simulink model "primary"  (R2017b)
settings: Solver=VariableStepAuto  StartTime=0.0  StopTime=10.0  RelTol=1e-3
model workspace (MAT data in the model file):
  Cf = 0
  F = 0
  Kic = 0
  Kiv = 0
  Kpc = 0
  Kpv = 0
  Lf = 0
  Vn = 0
  fn = 0
  m = 0
  n = 0
  wn = 0
libraries: powerlib x13, powerlib_meascontrol x5, simulink x4, pePowerMeasurement x1
settings Model: Creator=xx  LastModifiedBy=ongun

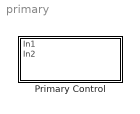
== system primary ==
  Primary Control : Subsystem

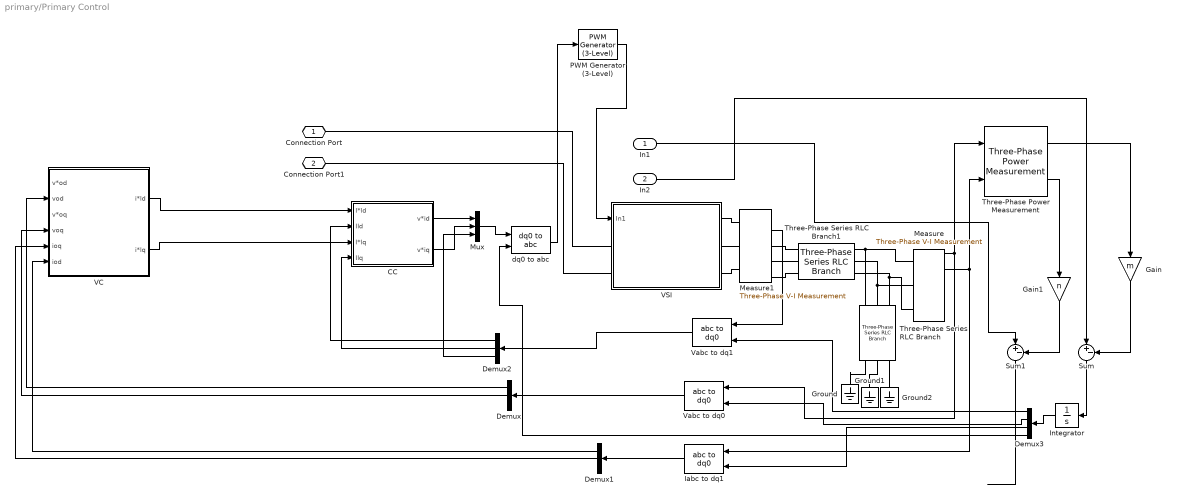
== system primary/Primary Control ==
  In1 : Inport
  In2 : Inport  Port=2
  CC : Subsystem
  Demux : Demux  Outputs=3
  Demux1 : Demux  Outputs=3
  Demux2 : Demux  Outputs=3
  Demux3 : Demux
  Gain : Gain  Gain=m
  Gain1 : Gain  Gain=n
  Ground : powerlib/Elements/Ground  LConnTagsString=a
  Ground1 : powerlib/Elements/Ground  LConnTagsString=a
  Ground2 : powerlib/Elements/Ground  LConnTagsString=a
  Iabc to dq1 : powerlib_meascontrol/Transformations/abc to dq0  Alignment=90 degrees behind phase A axis
  Integrator : Integrator
  Measure : powerlib/Measurements/Three-Phase V-I Measurement  VoltageMeasurement=phase-to-ground  SetLabelV=off  LabelV=V1  Vpu=off  VpuLL=off  CurrentMeasurement=yes  SetLabelI=off  LabelI=I1  Ipu=off  Pbase=5.5e3  Vbase=385  OutputType=Magnitude  PhasorSimulation=off  PSBequivalent=0
  Measure1 : powerlib/Measurements/Three-Phase V-I Measurement  VoltageMeasurement=phase-to-ground  SetLabelV=off  LabelV=V1  Vpu=off  VpuLL=off  CurrentMeasurement=yes  SetLabelI=off  LabelI=I1  Ipu=off  Pbase=5.5e3  Vbase=385  OutputType=Magnitude  PhasorSimulation=off  PSBequivalent=0
  Mux : Mux  Inputs=3
  PWM Generator (3-Level) : powerlib_meascontrol/Pulse & Signal Generators/PWM Generator (3-Level)  ModulatorType=Three-phase bridge (12 pulses)  ModulatorMode=Unsynchronized  nF=27  Fc=27*60  ModulatingSignals=off  m=0.8  Freq=60  Phase=0  Ts=0
      settings: SourceProductName=Simscape Power Systems  SourceProductBaseCode=PS
  Sum : Sum  Inputs=|+-
  Sum1 : Sum  Inputs=|+-
  Three-Phase Series RLC Branch : powerlib/Elements/Three-Phase Series RLC Branch  LConnTagsString=A|B|C  RConnTagsString=A|B|C  BranchType=C  Resistance=.1  Inductance=1e-3  Capacitance=6.85e-6  Measurements=None
  Three-Phase Series RLC Branch1 : powerlib/Elements/Three-Phase Series RLC Branch  LConnTagsString=A|B|C  RConnTagsString=A|B|C  BranchType=RL  Resistance=1  Inductance=1e-3  Capacitance=0  Measurements=None
  Three-Phase Power Measurement : pePowerMeasurement/Three-Phase Power Measurement  OverrideUsingVariant=Continuous  F=60  K=[0 1 2 3]  Seq=Positive  Ts=0
  VC : Subsystem
  VSI : Subsystem
  Vabc to dq0 : powerlib_meascontrol/Transformations/abc to dq0  Alignment=90 degrees behind phase A axis
  Vabc to dq1 : powerlib_meascontrol/Transformations/abc to dq0  Alignment=90 degrees behind phase A axis
  dq0 to abc : powerlib_meascontrol/Transformations/dq0 to abc  Alignment=90 degrees behind phase A axis
  Connection Port : PMIOPort  Port=1  Side=Left
  Connection Port1 : PMIOPort  Port=2  Side=Left
  wires:
  Demux/1 -> VC/2(vod)
  Demux/2 -> VC/4(voq)
  Measure/2 -> Three-Phase Power Measurement/2, Iabc to dq1/1
  Three-Phase Power Measurement/2 -> Gain1/1
  Demux2/2 -> CC/4(Ilq)
  In1/1 -> Sum1/1
  VC/1(i*ld) -> CC/1(I*ld)
  Measure1/2 -> Vabc to dq1/1
  In2/1 -> Sum/1
  Three-Phase Power Measurement/1 -> Gain/1
  Vabc to dq0/1 -> Demux/1
  Vabc to dq1/1 -> Demux2/1
  Gain1/1 -> Sum1/2
  Demux2/1 -> CC/2(Ild)
  Demux1/2 -> VC/5(ioq)
  Measure/1 -> Three-Phase Power Measurement/1, Vabc to dq0/1
  Gain/1 -> Sum/2
  Sum/1 -> Integrator/1
  VC/2("i*lq ") -> CC/3(I*lq)
  Demux1/1 -> VC/6(iod)
  Iabc to dq1/1 -> Demux1/1
  Sum1/1 -> ?
  CC/1(v*id) -> Mux/1
  CC/2("v*iq ") -> Mux/2
  Demux2/3 -> Mux/3
  Mux/1 -> dq0 to abc/1
  dq0 to abc/1 -> PWM Generator (3-Level)/1
  PWM Generator (3-Level)/1 -> VSI/1(In1)
  Integrator/1 -> Demux3/1
  Demux3/3 -> Iabc to dq1/2
  Demux3/2 -> Vabc to dq0/2
  Demux3/1 -> Vabc to dq1/2
  Demux3/4 -> dq0 to abc/2
  connections:
  VSI/RConn2 -- Measure1/LConn2
  VSI/RConn1 -- Measure1/LConn1
  VSI/RConn3 -- Measure1/LConn3
  Connection Port/RConn1 -- VSI/LConn1
  VSI/LConn2 -- Connection Port1/RConn1
  Three-Phase Series RLC Branch/LConn3 -- Measure/LConn3 -- Three-Phase Series RLC Branch1/RConn3
  Three-Phase Series RLC Branch1/RConn1 -- Measure/LConn1 -- Three-Phase Series RLC Branch/LConn1
  Three-Phase Series RLC Branch1/RConn2 -- Measure/LConn2 -- Three-Phase Series RLC Branch/LConn2
  Ground/LConn1 -- Three-Phase Series RLC Branch/RConn1
  Ground1/LConn1 -- Three-Phase Series RLC Branch/RConn2
  Ground2/LConn1 -- Three-Phase Series RLC Branch/RConn3
  Measure1/RConn1 -- Three-Phase Series RLC Branch1/LConn1
  Measure1/RConn2 -- Three-Phase Series RLC Branch1/LConn2
  Measure1/RConn3 -- Three-Phase Series RLC Branch1/LConn3

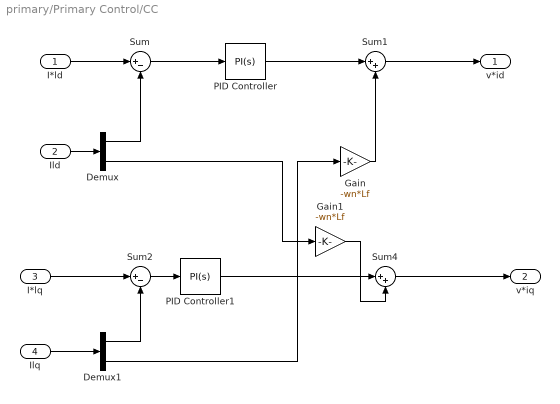
== system primary/Primary Control/CC ==
  I*ld : Inport
  Ild : Inport  Port=2
  I*lq : Inport  Port=3
  Ilq : Inport  Port=4
  Demux : Demux  Outputs=2
  Demux1 : Demux  Outputs=2
  Gain : Gain  Gain=-wn*Lf
  Gain1 : Gain  Gain=-wn*Lf
  PID Controller : simulink/Continuous/PID Controller  Controller=PI  TimeDomain=Continuous-time  SampleTime=-1  IntegratorMethod=Forward Euler  FilterMethod=Forward Euler  Form=Parallel  UseFilter=on  ControllerParametersSource=internal  P=Kpc  I=Kic  D=0  N=100  InitialConditionSource=internal  InitialConditionForIntegrator=0  InitialConditionForFilter=0  ExternalReset=none  LimitOutput=off  UpperSaturationLimit=inf  LowerSaturationLimit=-inf  LinearizeAsGain=on  AntiWindupMode=none  Kb=1  TrackingMode=off  Kt=1  PParamMin=[]  PParamMax=[]  IParamMin=[]  IParamMax=[]  DParamMin=[]  DParamMax=[]  NParamMin=[]  NParamMax=[]  KbParamMin=[]  KbParamMax=[]  KtParamMin=[]  KtParamMax=[]  POutMin=[]  POutMax=[]  IOutMin=[]  IOutMax=[]  DOutMin=[]  DOutMax=[]  NOutMin=[]  NOutMax=[]  KbOutMin=[]  KbOutMax=[]  KtOutMin=[]  KtOutMax=[]  IntegratorOutMin=[]  IntegratorOutMax=[]  FilterOutMin=[]  FilterOutMax=[]  SumOutMin=[]  SumOutMax=[]  SumI1OutMin=[]  SumI1OutMax=[]  SumI2OutMin=[]  SumI2OutMax=[]  SumI3OutMin=[]  SumI3OutMax=[]  SumDOutMin=[]  SumDOutMax=[]  SaturationOutMin=[]  SaturationOutMax=[]  IntegratorContinuousStateAttributes=''  IntegratorStateMustResolveToSignalObject=off  IntegratorRTWStateStorageClass=Auto  FilterContinuousStateAttributes=''  FilterStateMustResolveToSignalObject=off  FilterRTWStateStorageClass=Auto  DifferentiatorICPrevScaledInput=0  DifferentiatorOutMin=[]  DifferentiatorOutMax=[]  InitialConditionSetting=State (most efficient)  FilterDiffOutCoefMin=[]  FilterDiffOutCoefMax=[]  SumDenOutMin=[]  SumDenOutMax=[]  SumNumOutMin=[]  SumNumOutMax=[]  ReciprocalOutMin=[]  ReciprocalOutMax=[]  DivideOutMin=[]  DivideOutMax=[]  TunerSelectOption=Transfer Function Based (PID Tuner App)
  PID Controller1 : simulink/Continuous/PID Controller  Controller=PI  TimeDomain=Continuous-time  SampleTime=-1  IntegratorMethod=Forward Euler  FilterMethod=Forward Euler  Form=Parallel  UseFilter=on  ControllerParametersSource=internal  P=Kpc  I=Kic  D=0  N=100  InitialConditionSource=internal  InitialConditionForIntegrator=0  InitialConditionForFilter=0  ExternalReset=none  LimitOutput=off  UpperSaturationLimit=inf  LowerSaturationLimit=-inf  LinearizeAsGain=on  AntiWindupMode=none  Kb=1  TrackingMode=off  Kt=1  PParamMin=[]  PParamMax=[]  IParamMin=[]  IParamMax=[]  DParamMin=[]  DParamMax=[]  NParamMin=[]  NParamMax=[]  KbParamMin=[]  KbParamMax=[]  KtParamMin=[]  KtParamMax=[]  POutMin=[]  POutMax=[]  IOutMin=[]  IOutMax=[]  DOutMin=[]  DOutMax=[]  NOutMin=[]  NOutMax=[]  KbOutMin=[]  KbOutMax=[]  KtOutMin=[]  KtOutMax=[]  IntegratorOutMin=[]  IntegratorOutMax=[]  FilterOutMin=[]  FilterOutMax=[]  SumOutMin=[]  SumOutMax=[]  SumI1OutMin=[]  SumI1OutMax=[]  SumI2OutMin=[]  SumI2OutMax=[]  SumI3OutMin=[]  SumI3OutMax=[]  SumDOutMin=[]  SumDOutMax=[]  SaturationOutMin=[]  SaturationOutMax=[]  IntegratorContinuousStateAttributes=''  IntegratorStateMustResolveToSignalObject=off  IntegratorRTWStateStorageClass=Auto  FilterContinuousStateAttributes=''  FilterStateMustResolveToSignalObject=off  FilterRTWStateStorageClass=Auto  DifferentiatorICPrevScaledInput=0  DifferentiatorOutMin=[]  DifferentiatorOutMax=[]  InitialConditionSetting=State (most efficient)  FilterDiffOutCoefMin=[]  FilterDiffOutCoefMax=[]  SumDenOutMin=[]  SumDenOutMax=[]  SumNumOutMin=[]  SumNumOutMax=[]  ReciprocalOutMin=[]  ReciprocalOutMax=[]  DivideOutMin=[]  DivideOutMax=[]  TunerSelectOption=Transfer Function Based (PID Tuner App)
  Sum : Sum  Inputs=|+-
  Sum1 : Sum  Inputs=|++
  Sum2 : Sum  Inputs=|+-
  Sum4 : Sum  Inputs=|++
  v*id : Outport
  "v*iq " : Outport  Port=2
  wires:
  I*ld/1 -> Sum/1
  Ild/1 -> Demux/1
  I*lq/1 -> Sum2/1
  PID Controller/1 -> Sum1/1
  Sum/1 -> PID Controller/1
  Sum2/1 -> PID Controller1/1
  PID Controller1/1 -> Sum4/1
  Gain/1 -> Sum1/2
  Demux/2 -> Gain1/1
  Demux/1 -> Sum/2
  Sum4/1 -> "v*iq "/1
  Ilq/1 -> Demux1/1
  Demux1/1 -> Sum2/2
  Demux1/2 -> Gain/1
  Gain1/1 -> Sum4/2
  Sum1/1 -> v*id/1

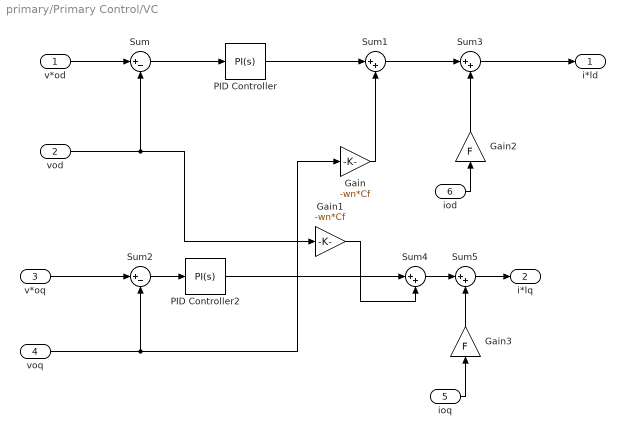
== system primary/Primary Control/VC ==
  v*od : Inport
  vod : Inport  Port=2
  v*oq : Inport  Port=3
  voq : Inport  Port=4
  ioq : Inport  Port=5
  iod : Inport  Port=6
  Gain : Gain  Gain=-wn*Cf
  Gain1 : Gain  Gain=-wn*Cf
  Gain2 : Gain  Gain=F
  Gain3 : Gain  Gain=F
  PID Controller : simulink/Continuous/PID Controller  Controller=PI  TimeDomain=Continuous-time  SampleTime=-1  IntegratorMethod=Forward Euler  FilterMethod=Forward Euler  Form=Parallel  UseFilter=on  ControllerParametersSource=internal  P=Kpv  I=Kiv  D=0  N=100  InitialConditionSource=internal  InitialConditionForIntegrator=0  InitialConditionForFilter=0  ExternalReset=none  LimitOutput=off  UpperSaturationLimit=inf  LowerSaturationLimit=-inf  LinearizeAsGain=on  AntiWindupMode=none  Kb=1  TrackingMode=off  Kt=1  PParamMin=[]  PParamMax=[]  IParamMin=[]  IParamMax=[]  DParamMin=[]  DParamMax=[]  NParamMin=[]  NParamMax=[]  KbParamMin=[]  KbParamMax=[]  KtParamMin=[]  KtParamMax=[]  POutMin=[]  POutMax=[]  IOutMin=[]  IOutMax=[]  DOutMin=[]  DOutMax=[]  NOutMin=[]  NOutMax=[]  KbOutMin=[]  KbOutMax=[]  KtOutMin=[]  KtOutMax=[]  IntegratorOutMin=[]  IntegratorOutMax=[]  FilterOutMin=[]  FilterOutMax=[]  SumOutMin=[]  SumOutMax=[]  SumI1OutMin=[]  SumI1OutMax=[]  SumI2OutMin=[]  SumI2OutMax=[]  SumI3OutMin=[]  SumI3OutMax=[]  SumDOutMin=[]  SumDOutMax=[]  SaturationOutMin=[]  SaturationOutMax=[]  IntegratorContinuousStateAttributes=''  IntegratorStateMustResolveToSignalObject=off  IntegratorRTWStateStorageClass=Auto  FilterContinuousStateAttributes=''  FilterStateMustResolveToSignalObject=off  FilterRTWStateStorageClass=Auto  DifferentiatorICPrevScaledInput=0  DifferentiatorOutMin=[]  DifferentiatorOutMax=[]  InitialConditionSetting=State (most efficient)  FilterDiffOutCoefMin=[]  FilterDiffOutCoefMax=[]  SumDenOutMin=[]  SumDenOutMax=[]  SumNumOutMin=[]  SumNumOutMax=[]  ReciprocalOutMin=[]  ReciprocalOutMax=[]  DivideOutMin=[]  DivideOutMax=[]  TunerSelectOption=Transfer Function Based (PID Tuner App)
  PID Controller2 : simulink/Continuous/PID Controller  Controller=PI  TimeDomain=Continuous-time  SampleTime=-1  IntegratorMethod=Forward Euler  FilterMethod=Forward Euler  Form=Parallel  UseFilter=on  ControllerParametersSource=internal  P=Kpv  I=Kiv  D=0  N=100  InitialConditionSource=internal  InitialConditionForIntegrator=0  InitialConditionForFilter=0  ExternalReset=none  LimitOutput=off  UpperSaturationLimit=inf  LowerSaturationLimit=-inf  LinearizeAsGain=on  AntiWindupMode=none  Kb=1  TrackingMode=off  Kt=1  PParamMin=[]  PParamMax=[]  IParamMin=[]  IParamMax=[]  DParamMin=[]  DParamMax=[]  NParamMin=[]  NParamMax=[]  KbParamMin=[]  KbParamMax=[]  KtParamMin=[]  KtParamMax=[]  POutMin=[]  POutMax=[]  IOutMin=[]  IOutMax=[]  DOutMin=[]  DOutMax=[]  NOutMin=[]  NOutMax=[]  KbOutMin=[]  KbOutMax=[]  KtOutMin=[]  KtOutMax=[]  IntegratorOutMin=[]  IntegratorOutMax=[]  FilterOutMin=[]  FilterOutMax=[]  SumOutMin=[]  SumOutMax=[]  SumI1OutMin=[]  SumI1OutMax=[]  SumI2OutMin=[]  SumI2OutMax=[]  SumI3OutMin=[]  SumI3OutMax=[]  SumDOutMin=[]  SumDOutMax=[]  SaturationOutMin=[]  SaturationOutMax=[]  IntegratorContinuousStateAttributes=''  IntegratorStateMustResolveToSignalObject=off  IntegratorRTWStateStorageClass=Auto  FilterContinuousStateAttributes=''  FilterStateMustResolveToSignalObject=off  FilterRTWStateStorageClass=Auto  DifferentiatorICPrevScaledInput=0  DifferentiatorOutMin=[]  DifferentiatorOutMax=[]  InitialConditionSetting=State (most efficient)  FilterDiffOutCoefMin=[]  FilterDiffOutCoefMax=[]  SumDenOutMin=[]  SumDenOutMax=[]  SumNumOutMin=[]  SumNumOutMax=[]  ReciprocalOutMin=[]  ReciprocalOutMax=[]  DivideOutMin=[]  DivideOutMax=[]  TunerSelectOption=Transfer Function Based (PID Tuner App)
  Sum : Sum  Inputs=|+-
  Sum{1,3..5} (4 alike) : Sum  Inputs=|++
  Sum2 : Sum  Inputs=|+-
  i*ld : Outport
  "i*lq " : Outport  Port=2
  wires:
  v*od/1 -> Sum/1
  v*oq/1 -> Sum2/1
  PID Controller/1 -> Sum1/1
  Sum/1 -> PID Controller/1
  Sum2/1 -> PID Controller2/1
  PID Controller2/1 -> Sum4/1
  Gain/1 -> Sum1/2
  vod/1 -> Sum/2, Gain1/1
  Sum4/1 -> Sum5/1
  voq/1 -> Gain/1, Sum2/2
  Gain1/1 -> Sum4/2
  ioq/1 -> Gain3/1
  Sum1/1 -> Sum3/1
  Sum3/1 -> i*ld/1
  iod/1 -> Gain2/1
  Sum5/1 -> "i*lq "/1
  Gain2/1 -> Sum3/2
  Gain3/1 -> Sum5/2

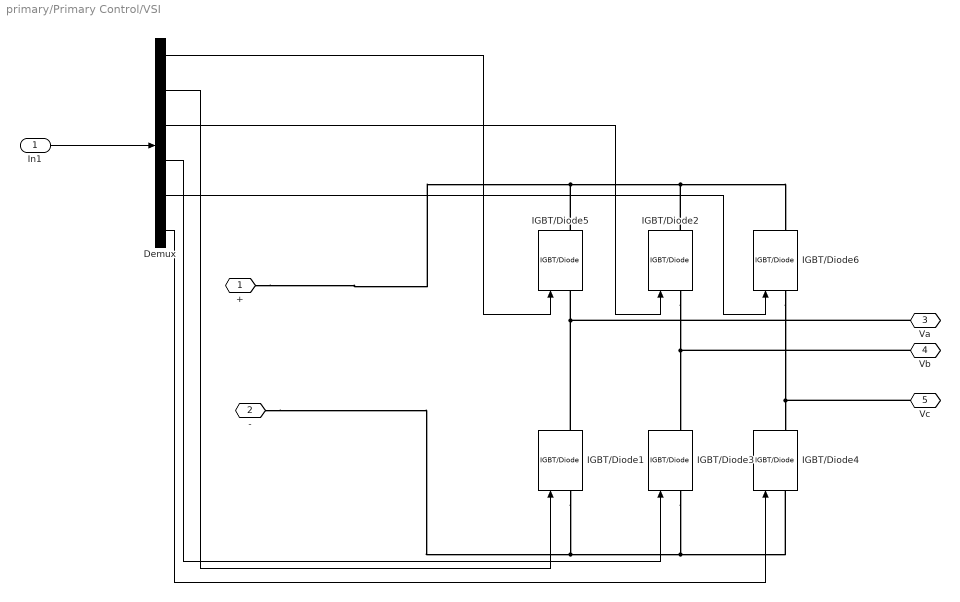
== system primary/Primary Control/VSI ==
  In1 : Inport
  Demux : Demux  Outputs=6
  IGBT/Diode{1..6} (6 alike) : powerlib/Power Electronics/IGBT//Diode  Ron=1e-3  Rs=1e5  Cs=inf  Measurements=on
  + : PMIOPort  Port=1  Side=Left
  - : PMIOPort  Port=2  Side=Left
  Va : PMIOPort  Port=3  Side=Right
  Vb : PMIOPort  Port=4  Side=Right
  Vc : PMIOPort  Port=5  Side=Right
  wires:
  Demux/1 -> IGBT/Diode5/1
  Demux/2 -> IGBT/Diode1/1
  Demux/3 -> IGBT/Diode2/1
  Demux/4 -> IGBT/Diode3/1
  Demux/5 -> IGBT/Diode6/1
  Demux/6 -> IGBT/Diode4/1
  In1/1 -> Demux/1
  connections:
  IGBT/Diode5/RConn1 -- IGBT/Diode2/RConn1 -- IGBT/Diode6/RConn1 -- +/RConn1
  Vb/RConn1 -- IGBT/Diode2/LConn1 -- IGBT/Diode3/RConn1
  IGBT/Diode6/LConn1 -- IGBT/Diode4/RConn1 -- Vc/RConn1
  IGBT/Diode1/LConn1 -- IGBT/Diode4/LConn1 -- IGBT/Diode3/LConn1 -- -/RConn1
  IGBT/Diode1/RConn1 -- IGBT/Diode5/LConn1 -- Va/RConn1
